simulink model "ES105A_StHlthSigNormn"  (R2013b)
settings: Solver=FixedStepDiscrete  SolverMode=SingleTasking  StartTime=0.0  StopTime=1  FixedStep=0.002  RelTol=1e-3
undefined symbols (not defined in the file): ARCHGLBPRM_FLOATZEROTHD_ULS_F32, CurrMeasCorrlnMaxErrCurr, CURRMOTSUMDIVBYZEROPROTNVAL_AMPR_F32, DIGTQDIVBYZEROPROTNVAL_HWNWTMTR_F32, DutyCycThermProtnDutyCycFildThd, EcuTMeasRngDiagcMax, EcuTMeasRngDiagcMin, EotLrngAuthyStrtLrn, FRICESTIMNDIVBYZEROPROTNVAL_HWNWTMTR_F32, HLTH0PERC_CNT_U08, HLTH100PERC_CNT_F32, HLTH100PERC_CNT_U08, HLTH50PERC_CNT_U08, HwTqCorrlnChATraSumSetFltThd, HwTqCorrlnChBTraSumSetFltThd, HWTQIDPTSIG_CNT_U08, MOTAG2MEAS_VALMAXERR_VOLTSQD_F32, MOTAG2MEAS_VALMINERR_VOLTSQD_F32, MOTAGCORRLN_MOTAGCORRLNERRTHD_MOTREVELEC_U0P16, MotDrvDiagcErrThd, MOTPOS2DIVBYZEROPROTNVAL2_VOLTSQD_F32, MOTPOS2DIVBYZEROPROTNVAL_VOLTSQD_F32, MOTPOSNERRDIVBYZEROPROTNVAL_MOTREV_U16, MOTPOSNERRZEROTHD_MOTREV_U0P16, NtcNr1, NtcSts1, PHAVLTGDIVBYZEROPROTNVAL_NANOSEC_F32, SigQlfr1, STHLTHSCAGFAC_CNT_F32, StHlthSigNormnAbsltMotPosDifStHlthDiagThd, StHlthSigNormnCurrMotSumStHlthDiagThd, StHlthSigNormnDigTqStHlthDiagThd, StHlthSigNormnDutyCycFltLimThd, StHlthSigNormnHiCtrlrT, StHlthSigNormnIdptSigStHlthSca, StHlthSigNormnLoCtrlrT, StHlthSigNormnMaxFricThd, StHlthSigNormnMinRackTrvlLim, StHlthSigNormnMotPosStHlthDiagThd, StHlthSigNormnMotVelCal, StHlthSigNormnPhaInfoStHlthDiagThd, StHlthSigNormnStHlthCorrlnErr, StHlthSigNormnStHlthCurrMotSum, StHlthSigNormnStHlthPhaInfo, StHlthSigNormnValMaxStHlthErr, StHlthSigNormnValMinStHlthErr, StHlthSigNormnWhlImbRejctnThd, SysGlbPrmMotPoleCnt, TSTHLTH0PERC_CNT_U08, u2, u3, u4, VLTGSTHLTH0PERC_CNT_U08
libraries: NxtrLim x39, simulink x33, NxtrAbslt x4
(part 1 of 10)
settings Model: Creator=PRAVEEND2  LastModifiedBy=DZ1YRM
settings SolverCC: AutoInsertRateTranBlk=on  InsertRTBMode=Always
settings DataIOCC: LimitDataPoints=off  SaveFormat=Structure  ReturnWorkspaceOutputs=on
settings OptimizationCC: BlockReduction=off  InlineParams=on  ZeroExternalMemoryAtStartup=off  ZeroInternalMemoryAtStartup=off  OptimizeModelRefInitCode=on  LifeSpan=1
settings DebuggingCC: SignalInfNanChecking=error  SignalRangeChecking=warning  UnderspecifiedInitializationDetection=Simplified  SolverPrmCheckMsg=error  InheritedTsInSrcMsg=error  DiscreteInheritContinuousMsg=error  SingleTaskRateTransMsg=error  TasksWithSamePriorityMsg=error  SigSpecEnsureSampleTimeMsg=error  CheckMatrixSingularityMsg=error  ParameterUnderflowMsg=error  ParameterPrecisionLossMsg=error  ParameterTunabilityLossMsg=error  FixptConstUnderflowMsg=warning  FixptConstOverflowMsg=warning  VectorMatrixConversionMsg=error  SignalLabelMismatchMsg=error  UnconnectedInputMsg=error  UnconnectedOutputMsg=error  UnconnectedLineMsg=error  SFcnCompatibilityMsg=error  UniqueDataStoreMsg=warning  BusObjectLabelMismatch=error  RootOutportRequireBusObject=error  AssertControl=DisableAll  ModelReferenceIOMsg=error  ModelReferenceVersionMismatchMessage=warning  ModelReferenceIOMismatchMessage=error  ModelReferenceCSMismatchMessage=warning  ModelReferenceDataLoggingMessage=error  StateNameClashWarn=warning  StrictBusMsg=ErrorOnBusTreatedAsVector  NonBusSignalsTreatedAsBus=error  SFUnexpectedBacktrackingDiag=error  SFInvalidInputDataAccessInChartInitDiag=error  SFNoUnconditionalDefaultTransitionDiag=error  SFTransitionOutsideNaturalParentDiag=error  SFUnconditionalTransitionShadowingDiag=error  SFUndirectedBroadcastEventsDiag=error
settings ModelReferenceCC: ModelReferenceNumInstancesAllowed=Single
settings RTWCC: SystemTargetFile=autosar.tlc  GenCodeOnly=on  TemplateMakefile=ert_default_tmf  Description=AUTOSAR  GenerateReport=on  ProcessScript=autosar_make_rtw_hook  LaunchReport=on
settings CodeAppCC: GenerateComments=off  IgnoreCustomStorageClasses=off  CustomSymbolStrType=$N$R$M  CustomSymbolStrBlkIO=$N$M  SimulinkBlockComments=off
settings STFCustomTargetCC: ParMdlRefBuildCompliant=on  CompOptLevelCompliant=on  IncludeMdlTerminateFcn=off  CombineOutputUpdateFcns=on  SuppressErrorStatus=on  ERTFirstTimeCompliant=on  ERTCustomFileBanners=on  SupportNonFinite=off  SupportComplex=off  SupportContinuousTime=off  SupportNonInlinedSFcns=off  MATLABClassNameForMDSCustomization=Simulink.SoftwareTarget.ERTCustomization  AutosarCompliant=on  GRTInterface=off  SystemTargetFile=autosar.tlc
settings ERTTargetCC: CodeReplacementLibrary=ANSI_C  ConcurrentExecutionCompliant=off  IncludeMdlTerminateFcn=off  SuppressErrorStatus=on  SupportNonFinite=off  SupportComplex=off  ModelStepFunctionPrototypeControlCompliant=off  CPPClassGenCompliant=off  AutosarCompliant=on  InlinedParameterPlacement=NonHierarchical  ERTCustomFileTemplate=example_file_process.tlc  EnableUserReplacementTypes=on

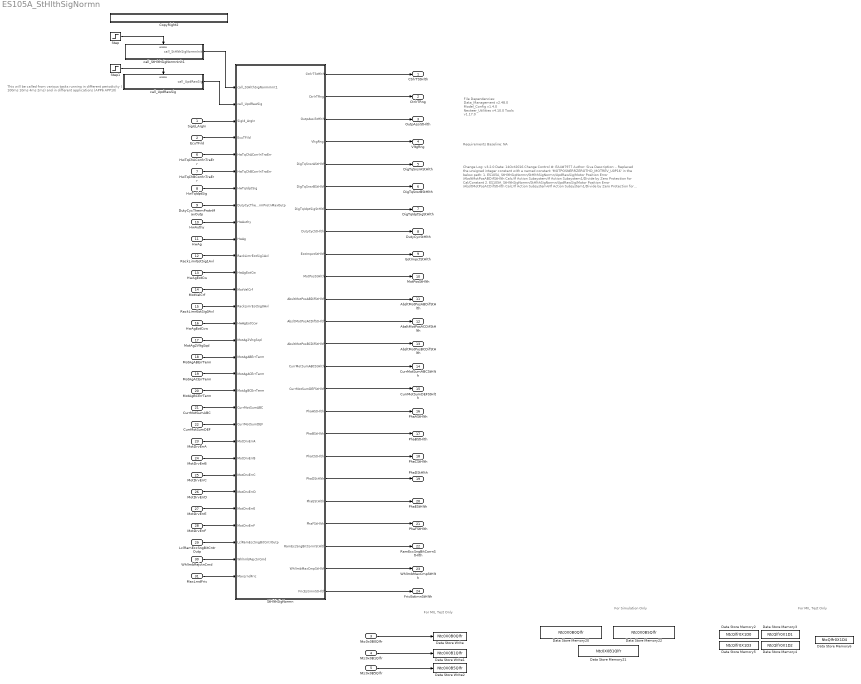
== system ES105A_StHlthSigNormn ==
  note: This will be called from various tasks running in different periodicity
      | ( 100ms 10ms 4ms 2ms) and in different applications (APP6 APP10)
  note: File Dependencies:
      |
      | Data_Management v2.48.0
      | Model_Config v1.4.0
      | Nexteer_Utilities v4.10.0
      | Tools v1.17.0
  note: Requirements Baseline: NA
  note: Change Log:
      |
      | v3.2.0
      | Date: 14Oct2016
      | Change Control #: EA4#7977
      | Author: Siva
      | Description:
      | - Replaced the unsigned integer constant with a named constant 'MOTPOSNERRZEROTHD_MOTREV_U0P16' in the below path:
      |         1. ES105A_StHlthSigNormn/StHlthSigNormn/UpdRawSig/Motor Position Error /AbsltMotPosABDifStHlth Calc/If Action
      |                Subsystem/If Action Subsystem1/Divide by Zero Protection for Cal/Constant
      |         2. ES105A_StHlthSigNormn/StHlthSigNormn/UpdRawSig/Motor Position Error /AbsltMotPosACDifStHlth Calc/If Action
      |                Subsystem4/If Action Subsystem1/Divide by Zero Protection for Cal/Constant1
      |         3. ES105A_StHlthSigNormn/StHlthSigNormn/UpdRawSig/Motor Position Error /AbsltMotPosBCDifStHlth Calc/If Action
      |                Subsystem8/If Action Subsystem1/Divide by Zero Protection for Cal/Constant1
      |
      | v3.1.0
      | Date: 28Sep2016
      | Change Control #: EA4#7764
      | Author: Siva
      | Description:
      | - Updated EOLFric (IRV signal) data dictionary information by swapping the ReadIn & WrittenIn attribute information.
      | - Updated Friction Estimation logic by performing all calculations in floating point mode and then converting it back to uint8 at the end.
      | - Removed extra saturation block present in the path(ES105A_StHlthSigNormn/StHlthSigNormn/UpdRawSig/Friction Estimation/LimStat_u2)
      |   as we have another saturation in the upstream logic.
      | - Replaced  'HLTH100PERC_CNT_U08' with a 'HLTH100PERC_CNT_F32' in both model & code.
      | - Replaced 'FRICESTSTHLTHLOLI_CNT_U08' & 'FRICESTSTHLTHHILI_CNT_U08' with 'FRICESTSTHLTHLOLI_CNT_F32' & 'FRICESTSTHLTHHILI_CNT_F32'
      |   in both model & code.
      | - Replaced numerical constant '1' of type 'uit8' with a 'float32' type.
      |
      | v3.0.0
      | Date: 23Sep2016
      | Change Control #: EA4#7256, EA4#7261, EA4#7303
      | Author: Siva
      | Description:
      | - Added Default labels to switch blocks in the below path:
      |        - ES105A_StHlthSigNormn/StHlthSigNormn/UpdRawSig/Switch Case1
      |        - ES105A_StHlthSigNormn/StHlthSigNormn/UpdRawSig/Digital Torque Sensor /Switch Case1
      |        - ES105A_StHlthSigNormn/StHlthSigNormn/UpdRawSig/Motor Position Error /Switch Case1
      |        - ES105A_StHlthSigNormn/StHlthSigNormn/UpdRawSig/Current Error/Switch Case1
      |        - ES105A_StHlthSigNormn/StHlthSigNormn/UpdRawSig/Phase Voltage Verification/Switch Case1
      | - Two New Outputs (WhlImbMaxCmpStHlth, FricEstimnStHlth) were added to model as well as DD.
      | - Two new Inputs (MaxLrndFric, WhlImbRejctnCmd) were added to to model and DD.
      |
      |
      |
      | v2.2.0
      | Date: 30Jun2016
      | Change Control #: EA4#5772, EA4#6242
      | Author: Siva, Mark Norman
      | Description:
      | - Added Saturation blocks to limit the Output value between [0 255] in all the below mentioned subsystems.
      |              -  Current Error
      |              -  Digital Torque Sensor
      |              -  Motor Position
      |              -  Motor Position Error
      |              -  Phase Voltage Verification
      | - Added Divide By Zero Protection blocks to limit the Output value between [0 255] in all the below mentioned subsystems.
      |              -  Motor Position
      | - Removed Default case from switch blocks in all the below mentioned subsystems.
      |              -  Current Error
      |              -  Digital Torque Sensor
      |              -  Motor Position Error
      |              -  Phase Voltage Verification
      |
      | Ver 2.1.0
      | DRW: Keyur G(KPIT)
      | Date:04-May-2016
      | CR- EA4#5550
      | -Default case added in switch cases to avoid simulation warnings
      | -Saturated input given to NTC status.
      | -Names of subsystems changed as per the requirement document.
      | -Name of signal 'VltgSqd' is changed to 'MotAg2VltgSqd' as it is an output from FDD ES241A. This change is done in model and .m file
      | - MotAgCorrlnErrThd and MOTAGCORRLN_MOTAGCORRLNERRTHD_MOTREVELEC_U0P16.LongName corrected
      | - Data type of Cal 'StHlthSigNormnStHlthCorrlnErr' is changed to u0p16 and 'StHlthSigNormnStHlthPhaInfo' is changed as float32
      | - Units of Cal StHlthSigNormnStHlthPhaInfo changed to 'NanoSec'
      | - Following constants have been added to replace magic numbers used for divide by zero protection logic
      | - DIGTQDIVBYZEROPROTNVAL_HWNWTMTR_F32, MOTPOSNERRDIVBYZEROPROTNVAL_MOTREV_U16, CURRMOTSUMDIVBYZEROPROTNVAL_AMPR_F32, PHAVLTGDIVBYZEROPROTNVAL_NANOSEC_F32
      | - Implementation added of PIM write and read for all NTC Sts calculations in Model and .m file.
      | - HUNDRED_CNT_U08 is changed to STHLTHSCAGFAC_CNT_F32.
      | - Removed Initialization of outputs from 'Init' function. Updated 'EngInit' and 'WrittenIn' field of all outputs with respective init value in Data Dict.
      | - Inside Digital Torque sensor Promotion of 1 is changed to Float32 in the below mentioned path:
      | 1).ES105A_StHlthSigNormn/StHlthSigNormn/UpdRawSig/Digital Torque Sensor /DigTqSnsrAStHlth Calc/If Action Subsystem1
      | 2) ES105A_StHlthSigNormn/StHlthSigNormn/UpdRawSig/Digital Torque Sensor /DigTqSnsrBStHlth Calc/If Action Subsystem3
      | - Inside EOT Impact Counter : HwAg comparion against zero is corrected to 'ARCHGLBPRM_FLOATZEROTHD_ULS_F32'
      | - Inside Motor Position Error in all cases: Divide-by-zero error protection logic Check against ARCHGLBPRM_FLOATZEROTHD_ULS_F32 is changed to zero.
      | - Initial output is kept hundred for all state health output port for all cases.
      | -Inside init subsystem, State Health PIM's are assigned with HLTH100PERC_CNT_U08 added
      |
      | Ver 2.0.0
      | DRW: Keyur G /Muragesh Asundi (KPIT)
      | Date:26-Apr-2016
      | CR- EA4#5550
      | -Design update as per new Requirements
      | -Constants for 0, 50,100 State of health is defined instead for having different constants for different State of health signals.
      | - Changes are marked with Red foreground color
      |
      | Ver 1.1.0
      | DRW:Praveen Devaraj(KPIT)
      | Date:11-Feb-2016
      | CR- EA4#3804
      | - Removed the PIM variable Intialization from Init function
      | -The Range limiter block placed outside the Init and server runnable is
      |   removed.Now it is placed inside the server runnable.
      | - In DD, EngValue are changed for EcuTMeasRngDiagcMax = 145,
      |   EcuTMeasRngDiagcMin = -45,StHlthSigNormnHiCtrlrT = 140
      |   StHlthSigNormnLoCtrlrT = -40.
      |
      | Ver: 1.0.0
      | DRW:Shradha Manusmare/Praveen Devaraj(KPIT)
      | Date:08-Feb-2016
      | CR- EA4#3077
      | - EA4 Initial Version
  note: For MIL Test Only
  note: For MIL Test Only
  note: For Simulation Only
  SigId_ArgIn : Inport
  EcuTFild : Inport  Port=2
  Ntc0x0B0Qlfr : Inport  Port=3
  Ntc0x0B1Qlfr : Inport  Port=4
  Ntc0x0B5Qlfr : Inport  Port=5
  HwTqChACorrlnTraErr : Inport  Port=6
  HwTqChBCorrlnTraErr : Inport  Port=7
  HwTqIdptSig : Inport  Port=8
  DutyCycThermProtnMaxOutp : Inport  Port=9
  HwAuthy : Inport  Port=10
  HwAg : Inport  Port=11
  RackLimrEotSig1Avl : Inport  Port=12
  HwAgEotCw : Inport  Port=13
  MotVelCrf : Inport  Port=14
  RackLimrEotSig0Avl : Inport  Port=15
  HwAgEotCcw : Inport  Port=16
  MotAg2VltgSqd : Inport  Port=17
  MotAgABErrTerm : Inport  Port=18
  MotAgACErrTerm : Inport  Port=19
  MotAgBCErrTerm : Inport  Port=20
  CurrMotSumABC : Inport  Port=21
  CurrMotSumDEF : Inport  Port=22
  MotDrvErrA : Inport  Port=23
  MotDrvErrB : Inport  Port=24
  MotDrvErrC : Inport  Port=25
  MotDrvErrD : Inport  Port=26
  MotDrvErrE : Inport  Port=27
  MotDrvErrF : Inport  Port=28
  LclRamEccSngBitCntrOutp : Inport  Port=29
  WhlImbRejctnCmd : Inport  Port=30
  MaxLrndFric : Inport  Port=31
  CopyRight2 : Subsystem  Description=|  mask(Copyright Information){none=on}
      | Copyright info block.                                               
      |                                                                     
      | Place copyright information at the top of every subsystem in design.
      mask prompts: none "No parameters"
      mask help: Place copyright information at the top of every subsystem in design.
      mask Display:
      | NxtrConf = 'Nexteer Confidential';
      | 
      | sys = bdroot; %handle for the current model ("system")
      | first = get_param(sys,'Created');
      | first = first(end-3:end);  %year is last four digits
      | 
      | last = get_param(sys,'LastModifiedDate');
      | if isempty(last)
      |     last = datestr(now,'yyyy');
      | else
      |     last = last(end-3:end);
      | end
      | 
      | if strcmp(first,last)
      |     fprintf('%s -- Copyright %s Nexteer',NxtrConf,first)
      | else
      |     fprintf('%s -- %s%s- %s Nexteer',NxtrConf,char(169),first,last)
      | end
  Data Store Memory2 : DataStoreMemory  DataStoreName=NtcQlfr0X1D0
  Data Store Memory20 : DataStoreMemory  DataStoreName=Ntc0X0B0Qlfr  InitialValue=SigQlfr1.SIGQLFR_NORES  OutDataTypeStr=Enum: SigQlfr1
      settings: LockScale=on
  Data Store Memory21 : DataStoreMemory  DataStoreName=Ntc0X0B1Qlfr  InitialValue=SigQlfr1.SIGQLFR_NORES  OutDataTypeStr=Enum: SigQlfr1
  Data Store Memory22 : DataStoreMemory  DataStoreName=Ntc0X0B5Qlfr  InitialValue=SigQlfr1.SIGQLFR_NORES  OutDataTypeStr=Enum: SigQlfr1
  Data Store Memory3 : DataStoreMemory  DataStoreName=NtcQlfr0X1D1
  Data Store Memory4 : DataStoreMemory  DataStoreName=NtcQlfr0X1D2
  Data Store Memory5 : DataStoreMemory  DataStoreName=NtcQlfr0X1D3
  Data Store Memory6 : DataStoreMemory  DataStoreName=NtcQlfr0X1D4
  Data Store Write : DataStoreWrite  DataStoreName=Ntc0X0B0Qlfr
  Data Store Write1 : DataStoreWrite  DataStoreName=Ntc0X0B1Qlfr
  Data Store Write2 : DataStoreWrite  DataStoreName=Ntc0X0B5Qlfr
  StHlthSigNormn : Subsystem  RequirementInfo={'linktype_rmi_doors' '0001022c (/ESG Group/FDD Module Requirements/EA4 Specific/ES105A_StHlthSigNormn)' '#ES105A_6' 'true' 'REQ: ES105A_6' '' ; 'linktype_rmi_doors' '0001022c (/ESG Group/FDD Module Requirements/EA4 Specific/ES105A_StHlthSigNormn)' '#ES105A_7' 'true' 'REQ: ES105A_7' '' } %GIDa_6ff4320a_4d8a_4175_a33b_02dee4a007dc
  Step : Step  Before=1  After=0  SampleTime=0.002
  Step1 : Step  SampleTime=0.002
  call_StHlthSigNormnInit1 : Subsystem  TreatAsAtomicUnit=on
  call_UpdRawSig : Subsystem  RequirementInfo={'linktype_rmi_doors' '0001022c (/ESG Group/FDD Module Requirements/EA4 Specific/ES105A_StHlthSigNormn)' '#ES105A_8' 'true' 'REQ: ES105A_8' '' } %GIDa_42dfbf7d_1872_4f82_ac73_93b666af75d7  TreatAsAtomicUnit=on
  CtrlrTStHlth : Outport
  CtrlrTRng : Outport  Port=2
  OutpAssiStHlth : Outport  Port=3
  VltgRng : Outport  Port=4
  DigTqSnsrAStHlth : Outport  Port=5
  DigTqSnsrBStHlth : Outport  Port=6
  DigTqIdptSigStHlth : Outport  Port=7
  DutyCycStHlth : Outport  Port=8
  EotImpctStHlth : Outport  Port=9
  MotPosStHlth : Outport  Port=10
  AbsltMotPosABDifStHlth : Outport  Port=11
  AbsltMotPosACDifStHlth : Outport  Port=12
  AbsltMotPosBCDifStHlth : Outport  Port=13
  CurrMotSumABCStHlth : Outport  Port=14
  CurrMotSumDEFStHlth : Outport  Port=15
  PhaAStHlth : Outport  Port=16
  PhaBStHlth : Outport  Port=17
  PhaCStHlth : Outport  Port=18
  PhaDStHlth : Outport  Port=19
  PhaEStHlth : Outport  Port=20
  PhaFStHlth : Outport  Port=21
  RamEccSngBitCorrnStHlth : Outport  Port=22
  WhlImbMaxCmpStHlth : Outport  Port=23
  FricEstimnStHlth : Outport  Port=24
  wires:
  Step/1 -> call_StHlthSigNormnInit1/Enable
  call_StHlthSigNormnInit1/1(call_StHlthSigNormnInit1) -> StHlthSigNormn/1(call_StHlthSigNormnInit1)
  call_UpdRawSig/1(call_UpdRawSig) -> StHlthSigNormn/2(call_UpdRawSig)
  Step1/1 -> call_UpdRawSig/Enable
  SigId_ArgIn/1 -> StHlthSigNormn/3(SigId_ArgIn)
  EcuTFild/1 -> StHlthSigNormn/4(EcuTFild)
  Ntc0x0B0Qlfr/1 -> Data Store Write/1
  Ntc0x0B1Qlfr/1 -> Data Store Write1/1
  Ntc0x0B5Qlfr/1 -> Data Store Write2/1
  DutyCycThermProtnMaxOutp/1 -> StHlthSigNormn/8(DutyCycThermProtnMaxOutp)
  HwTqChACorrlnTraErr/1 -> StHlthSigNormn/5(HwTqChACorrlnTraErr)
  HwTqIdptSig/1 -> StHlthSigNormn/7(HwTqIdptSig)
  HwTqChBCorrlnTraErr/1 -> StHlthSigNormn/6(HwTqChBCorrlnTraErr)
  HwAuthy/1 -> StHlthSigNormn/9(HwAuthy)
  HwAg/1 -> StHlthSigNormn/10(HwAg)
  RackLimrEotSig1Avl/1 -> StHlthSigNormn/11(RackLimrEotSig1Avl)
  HwAgEotCw/1 -> StHlthSigNormn/12(HwAgEotCw)
  MotVelCrf/1 -> StHlthSigNormn/13(MotVelCrf)
  RackLimrEotSig0Avl/1 -> StHlthSigNormn/14(RackLimrEotSig0Avl)
  HwAgEotCcw/1 -> StHlthSigNormn/15(HwAgEotCcw)
  MotAg2VltgSqd/1 -> StHlthSigNormn/16(MotAg2VltgSqd)
  MotAgABErrTerm/1 -> StHlthSigNormn/17(MotAgABErrTerm)
  MotAgACErrTerm/1 -> StHlthSigNormn/18(MotAgACErrTerm)
  MotAgBCErrTerm/1 -> StHlthSigNormn/19(MotAgBCErrTerm)
  CurrMotSumABC/1 -> StHlthSigNormn/20(CurrMotSumABC)
  LclRamEccSngBitCntrOutp/1 -> StHlthSigNormn/28(LclRamEccSngBitCntrOutp)
  MotDrvErrF/1 -> StHlthSigNormn/27(MotDrvErrF)
  MotDrvErrE/1 -> StHlthSigNormn/26(MotDrvErrE)
  MotDrvErrD/1 -> StHlthSigNormn/25(MotDrvErrD)
  MotDrvErrC/1 -> StHlthSigNormn/24(MotDrvErrC)
  MotDrvErrA/1 -> StHlthSigNormn/22(MotDrvErrA)
  CurrMotSumDEF/1 -> StHlthSigNormn/21(CurrMotSumDEF)
  MotDrvErrB/1 -> StHlthSigNormn/23(MotDrvErrB)
  MaxLrndFric/1 -> StHlthSigNormn/30(MaxLrndFric)
  WhlImbRejctnCmd/1 -> StHlthSigNormn/29(WhlImbRejctnCmd)
  StHlthSigNormn/22(RamEccSngBitCorrnStHlth) -> RamEccSngBitCorrnStHlth/1
  StHlthSigNormn/21(PhaFStHlth) -> PhaFStHlth/1
  StHlthSigNormn/20(PhaEStHlth) -> PhaEStHlth/1
  StHlthSigNormn/23(WhlImbMaxCmpStHlth) -> WhlImbMaxCmpStHlth/1
  StHlthSigNormn/24(FricEstimnStHlth) -> FricEstimnStHlth/1
  StHlthSigNormn/19(PhaDStHlth) -> PhaDStHlth/1
  StHlthSigNormn/18(PhaCStHlth) -> PhaCStHlth/1
  StHlthSigNormn/17(PhaBStHlth) -> PhaBStHlth/1
  StHlthSigNormn/16(PhaAStHlth) -> PhaAStHlth/1
  StHlthSigNormn/15(CurrMotSumDEFStHlth) -> CurrMotSumDEFStHlth/1
  StHlthSigNormn/14(CurrMotSumABCStHlth) -> CurrMotSumABCStHlth/1
  StHlthSigNormn/13(AbsltMotPosBCDifStHlth) -> AbsltMotPosBCDifStHlth/1
  StHlthSigNormn/12(AbsltMotPosACDifStHlth) -> AbsltMotPosACDifStHlth/1
  StHlthSigNormn/11(AbsltMotPosABDifStHlth) -> AbsltMotPosABDifStHlth/1
  StHlthSigNormn/10(MotPosStHlth) -> MotPosStHlth/1
  StHlthSigNormn/9(EotImpctStHlth) -> EotImpctStHlth/1
  StHlthSigNormn/8(DutyCycStHlth) -> DutyCycStHlth/1
  StHlthSigNormn/7(DigTqIdptSigStHlth) -> DigTqIdptSigStHlth/1
  StHlthSigNormn/6(DigTqSnsrBStHlth) -> DigTqSnsrBStHlth/1
  StHlthSigNormn/5(DigTqSnsrAStHlth) -> DigTqSnsrAStHlth/1
  StHlthSigNormn/4(VltgRng) -> VltgRng/1
  StHlthSigNormn/3(OutpAssiStHlth) -> OutpAssiStHlth/1
  StHlthSigNormn/2(CtrlrTRng) -> CtrlrTRng/1
  StHlthSigNormn/1(CtrlrTStHlth) -> CtrlrTStHlth/1

== system ES105A_StHlthSigNormn/CopyRight2 ==

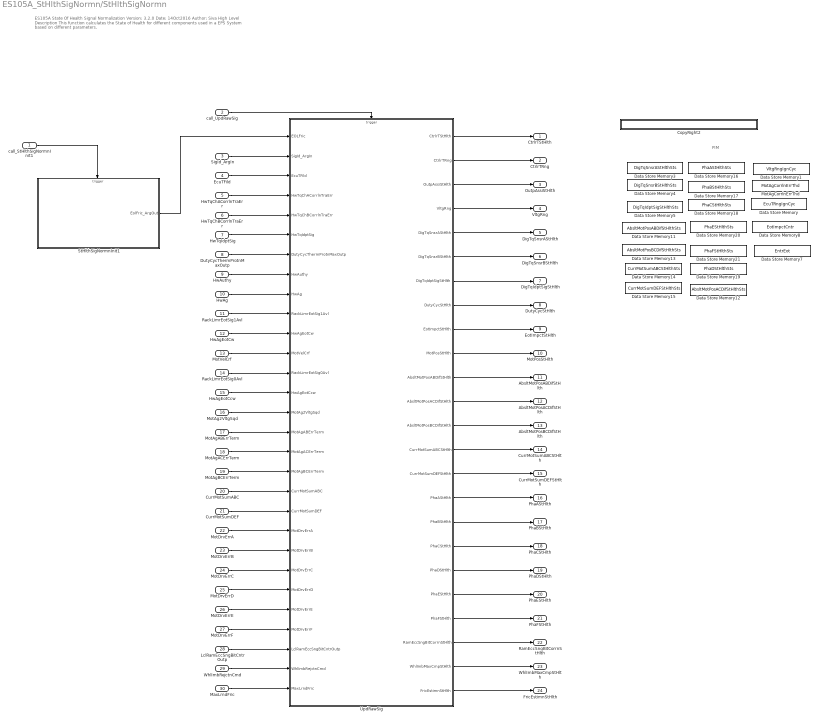
== system ES105A_StHlthSigNormn/StHlthSigNormn ==
  note: ES105A  State Of Health Signal Normalization
      |
      | Version: 3.2.0
      | Date: 14Oct2016
      |
      | Author: Siva
      |
      |
      | High Level Description
      |      This function calculates the State of Health for different components used in a EPS System based on different parameters.
  note: PIM
  call_StHlthSigNormnInit1 : Inport
  call_UpdRawSig : Inport  Port=2
  SigId_ArgIn : Inport  Port=3
  EcuTFild : Inport  RequirementInfo={'linktype_rmi_doors' '0001022c (/ESG Group/FDD Module Requirements/EA4 Specific/ES105A_StHlthSigNormn)' '#ES105A_14' 'true' 'REQ: ES105A_14' '' } %GIDa_49447a9e_c422_403c_bc64_e6d6f4ec146f  Port=4
  HwTqChACorrlnTraErr : Inport  Port=5
  HwTqChBCorrlnTraErr : Inport  Port=6
  HwTqIdptSig : Inport  Port=7
  DutyCycThermProtnMaxOutp : Inport  Port=8
  HwAuthy : Inport  Port=9
  HwAg : Inport  Port=10
  RackLimrEotSig1Avl : Inport  Port=11
  HwAgEotCw : Inport  Port=12
  MotVelCrf : Inport  Port=13
  RackLimrEotSig0Avl : Inport  Port=14
  HwAgEotCcw : Inport  Port=15
  MotAg2VltgSqd : Inport  Port=16
  MotAgABErrTerm : Inport  Port=17
  MotAgACErrTerm : Inport  Port=18
  MotAgBCErrTerm : Inport  Port=19
  CurrMotSumABC : Inport  Port=20
  CurrMotSumDEF : Inport  Port=21
  MotDrvErrA : Inport  Port=22
  MotDrvErrB : Inport  Port=23
  MotDrvErrC : Inport  Port=24
  MotDrvErrD : Inport  Port=25
  MotDrvErrE : Inport  Port=26
  MotDrvErrF : Inport  Port=27
  LclRamEccSngBitCntrOutp : Inport  Port=28
  WhlImbRejctnCmd : Inport  Port=29
  MaxLrndFric : Inport  Port=30
  CopyRight2 : Subsystem  Description=|  mask(Copyright Information){none=on}
      | Copyright info block.                                               
      |                                                                     
      | Place copyright information at the top of every subsystem in design.
      mask prompts: none "No parameters"
      mask help: Place copyright information at the top of every subsystem in design.
      mask Display:
      | NxtrConf = 'Nexteer Confidential';
      | 
      | sys = bdroot; %handle for the current model ("system")
      | first = get_param(sys,'Created');
      | first = first(end-3:end);  %year is last four digits
      | 
      | last = get_param(sys,'LastModifiedDate');
      | if isempty(last)
      |     last = datestr(now,'yyyy');
      | else
      |     last = last(end-3:end);
      | end
      | 
      | if strcmp(first,last)
      |     fprintf('%s -- Copyright %s Nexteer',NxtrConf,first)
      | else
      |     fprintf('%s -- %s%s- %s Nexteer',NxtrConf,char(169),first,last)
      | end
  Data Store Memory : DataStoreMemory  DataStoreName=EcuTRngIgnCyc  StateMustResolveToSignalObject=on
  Data Store Memory1 : DataStoreMemory  DataStoreName=VltgRngIgnCyc  StateMustResolveToSignalObject=on
  Data Store Memory11 : DataStoreMemory  DataStoreName=AbsltMotPosABDifStHlthSts  ReadBeforeWriteMsg=warning  WriteAfterWriteMsg=warning  WriteAfterReadMsg=warning  StateMustResolveToSignalObject=on
  Data Store Memory12 : DataStoreMemory  DataStoreName=AbsltMotPosACDifStHlthSts  ReadBeforeWriteMsg=warning  WriteAfterWriteMsg=warning  WriteAfterReadMsg=warning  StateMustResolveToSignalObject=on
  Data Store Memory13 : DataStoreMemory  DataStoreName=AbsltMotPosBCDifStHlthSts  ReadBeforeWriteMsg=warning  WriteAfterWriteMsg=warning  WriteAfterReadMsg=warning  StateMustResolveToSignalObject=on
  Data Store Memory14 : DataStoreMemory  DataStoreName=CurrMotSumABCStHlthSts  ReadBeforeWriteMsg=warning  WriteAfterWriteMsg=warning  WriteAfterReadMsg=warning  StateMustResolveToSignalObject=on
  Data Store Memory15 : DataStoreMemory  DataStoreName=CurrMotSumDEFStHlthSts  ReadBeforeWriteMsg=warning  WriteAfterWriteMsg=warning  WriteAfterReadMsg=warning  StateMustResolveToSignalObject=on
  Data Store Memory16 : DataStoreMemory  DataStoreName=PhaAStHlthSts  ReadBeforeWriteMsg=warning  WriteAfterWriteMsg=warning  WriteAfterReadMsg=warning  StateMustResolveToSignalObject=on
  Data Store Memory17 : DataStoreMemory  DataStoreName=PhaBStHlthSts  ReadBeforeWriteMsg=warning  WriteAfterWriteMsg=warning  WriteAfterReadMsg=warning  StateMustResolveToSignalObject=on
  Data Store Memory18 : DataStoreMemory  DataStoreName=PhaCStHlthSts  ReadBeforeWriteMsg=warning  WriteAfterWriteMsg=warning  WriteAfterReadMsg=warning  StateMustResolveToSignalObject=on
  Data Store Memory19 : DataStoreMemory  DataStoreName=PhaDStHlthSts  ReadBeforeWriteMsg=warning  WriteAfterWriteMsg=warning  WriteAfterReadMsg=warning  StateMustResolveToSignalObject=on
  Data Store Memory20 : DataStoreMemory  DataStoreName=PhaEStHlthSts  ReadBeforeWriteMsg=warning  WriteAfterWriteMsg=warning  WriteAfterReadMsg=warning  StateMustResolveToSignalObject=on
  Data Store Memory21 : DataStoreMemory  DataStoreName=PhaFStHlthSts  ReadBeforeWriteMsg=warning  WriteAfterWriteMsg=warning  WriteAfterReadMsg=warning  StateMustResolveToSignalObject=on
  Data Store Memory3 : DataStoreMemory  DataStoreName=DigTqSnsrAStHlthSts  ReadBeforeWriteMsg=warning  WriteAfterWriteMsg=warning  WriteAfterReadMsg=warning  StateMustResolveToSignalObject=on
  Data Store Memory4 : DataStoreMemory  DataStoreName=DigTqSnsrBStHlthSts  ReadBeforeWriteMsg=warning  WriteAfterWriteMsg=warning  WriteAfterReadMsg=warning  StateMustResolveToSignalObject=on
  Data Store Memory5 : DataStoreMemory  DataStoreName=DigTqIdptSigStHlthSts  ReadBeforeWriteMsg=warning  WriteAfterWriteMsg=warning  WriteAfterReadMsg=warning  StateMustResolveToSignalObject=on
  Data Store Memory7 : DataStoreMemory  DataStoreName=EntrEot  ReadBeforeWriteMsg=warning  WriteAfterWriteMsg=warning  WriteAfterReadMsg=warning  StateMustResolveToSignalObject=on
  Data Store Memory8 : DataStoreMemory  DataStoreName=EotImpctCntr  ReadBeforeWriteMsg=warning  WriteAfterWriteMsg=warning  WriteAfterReadMsg=warning  InitialValue=[]  StateMustResolveToSignalObject=on
  MotAgCorrlnErrThd : DataStoreMemory  Priority=0  DataStoreName=MotAgCorrlnErrThd  StateMustResolveToSignalObject=on
  StHlthSigNormnInit1 : Subsystem  RequirementInfo={'linktype_rmi_doors' '0001022c (/ESG Group/FDD Module Requirements/EA4 Specific/ES105A_StHlthSigNormn)' '#ES105A_9' 'true' 'REQ: ES105A_9' '' } %GIDa_bead402a_6bb2_4a86_9345_52509e5d4e33  TreatAsAtomicUnit=on
  UpdRawSig : Subsystem
  CtrlrTStHlth : Outport  RequirementInfo={'linktype_rmi_doors' '0001022c (/ESG Group/FDD Module Requirements/EA4 Specific/ES105A_StHlthSigNormn)' '#ES105A_26' 'true' 'REQ: ES105A_26' '' } %GIDa_65c3929a_51bb_49c3_afb4_64b9773c7714
  CtrlrTRng : Outport  RequirementInfo={'linktype_rmi_doors' '0001022c (/ESG Group/FDD Module Requirements/EA4 Specific/ES105A_StHlthSigNormn)' '#ES105A_26' 'true' 'REQ: ES105A_26' '' } %GIDa_a95003b5_b445_43be_bc6a_73ebe3208c85  Port=2
  OutpAssiStHlth : Outport  RequirementInfo={'linktype_rmi_doors' '0001022c (/ESG Group/FDD Module Requirements/EA4 Specific/ES105A_StHlthSigNormn)' '#ES105A_27' 'true' 'REQ: ES105A_27' '' } %GIDa_e353623f_856a_448e_be29_9e3993fbb0c1  Port=3
  VltgRng : Outport  RequirementInfo={'linktype_rmi_doors' '0001022c (/ESG Group/FDD Module Requirements/EA4 Specific/ES105A_StHlthSigNormn)' '#ES105A_27' 'true' 'REQ: ES105A_27' '' } %GIDa_05a6fd54_b3c2_4a26_803e_604d93a16994  Port=4
  DigTqSnsrAStHlth : Outport  Port=5
  DigTqSnsrBStHlth : Outport  Port=6
  DigTqIdptSigStHlth : Outport  Port=7
  DutyCycStHlth : Outport  Port=8
  EotImpctStHlth : Outport  Port=9
  MotPosStHlth : Outport  Port=10
  AbsltMotPosABDifStHlth : Outport  Port=11
  AbsltMotPosACDifStHlth : Outport  Port=12
  AbsltMotPosBCDifStHlth : Outport  Port=13
  CurrMotSumABCStHlth : Outport  Port=14
  CurrMotSumDEFStHlth : Outport  Port=15
  PhaAStHlth : Outport  Port=16
  PhaBStHlth : Outport  Port=17
  PhaCStHlth : Outport  Port=18
  PhaDStHlth : Outport  Port=19
  PhaEStHlth : Outport  Port=20
  PhaFStHlth : Outport  Port=21
  RamEccSngBitCorrnStHlth : Outport  Port=22
  WhlImbMaxCmpStHlth : Outport  Port=23
  FricEstimnStHlth : Outport  Port=24
  wires:
  call_StHlthSigNormnInit1/1 -> StHlthSigNormnInit1/Trigger
  UpdRawSig/21(PhaFStHlth) -> PhaFStHlth/1
  UpdRawSig/20(PhaEStHlth) -> PhaEStHlth/1
  UpdRawSig/22(RamEccSngBitCorrnStHlth) -> RamEccSngBitCorrnStHlth/1
  UpdRawSig/24(FricEstimnStHlth) -> FricEstimnStHlth/1
  UpdRawSig/23(WhlImbMaxCmpStHlth) -> WhlImbMaxCmpStHlth/1
  UpdRawSig/19(PhaDStHlth) -> PhaDStHlth/1
  UpdRawSig/18(PhaCStHlth) -> PhaCStHlth/1
  UpdRawSig/17(PhaBStHlth) -> PhaBStHlth/1
  UpdRawSig/16(PhaAStHlth) -> PhaAStHlth/1
  UpdRawSig/15(CurrMotSumDEFStHlth) -> CurrMotSumDEFStHlth/1
  UpdRawSig/14(CurrMotSumABCStHlth) -> CurrMotSumABCStHlth/1
  UpdRawSig/13(AbsltMotPosBCDifStHlth) -> AbsltMotPosBCDifStHlth/1
  UpdRawSig/12(AbsltMotPosACDifStHlth) -> AbsltMotPosACDifStHlth/1
  UpdRawSig/11(AbsltMotPosABDifStHlth) -> AbsltMotPosABDifStHlth/1
  UpdRawSig/10(MotPosStHlth) -> MotPosStHlth/1
  UpdRawSig/9(EotImpctStHlth) -> EotImpctStHlth/1
  UpdRawSig/8(DutyCycStHlth) -> DutyCycStHlth/1
  UpdRawSig/7(DigTqIdptSigStHlth) -> DigTqIdptSigStHlth/1
  UpdRawSig/6(DigTqSnsrBStHlth) -> DigTqSnsrBStHlth/1
  UpdRawSig/5(DigTqSnsrAStHlth) -> DigTqSnsrAStHlth/1
  UpdRawSig/4(VltgRng) -> VltgRng/1
  UpdRawSig/3(OutpAssiStHlth) -> OutpAssiStHlth/1
  UpdRawSig/2(CtrlrTRng) -> CtrlrTRng/1
  UpdRawSig/1(CtrlrTStHlth) -> CtrlrTStHlth/1
  call_UpdRawSig/1 -> UpdRawSig/Trigger
  MotDrvErrC/1 -> UpdRawSig/23(MotDrvErrC)
  MotDrvErrB/1 -> UpdRawSig/22(MotDrvErrB)
  MotDrvErrD/1 -> UpdRawSig/24(MotDrvErrD)
  MotDrvErrA/1 -> UpdRawSig/21(MotDrvErrA)
  MotDrvErrE/1 -> UpdRawSig/25(MotDrvErrE)
  CurrMotSumDEF/1 -> UpdRawSig/20(CurrMotSumDEF)
  MotDrvErrF/1 -> UpdRawSig/26(MotDrvErrF)
  MaxLrndFric/1 -> UpdRawSig/29(MaxLrndFric)
  CurrMotSumABC/1 -> UpdRawSig/19(CurrMotSumABC)
  LclRamEccSngBitCntrOutp/1 -> UpdRawSig/27(LclRamEccSngBitCntrOutp)
  WhlImbRejctnCmd/1 -> UpdRawSig/28(WhlImbRejctnCmd)
  MotAgBCErrTerm/1 -> UpdRawSig/18(MotAgBCErrTerm)
  MotAgACErrTerm/1 -> UpdRawSig/17(MotAgACErrTerm)
  MotAgABErrTerm/1 -> UpdRawSig/16(MotAgABErrTerm)
  MotAg2VltgSqd/1 -> UpdRawSig/15(MotAg2VltgSqd)
  HwAgEotCcw/1 -> UpdRawSig/14(HwAgEotCcw)
  RackLimrEotSig0Avl/1 -> UpdRawSig/13(RackLimrEotSig0Avl)
  MotVelCrf/1 -> UpdRawSig/12(MotVelCrf)
  HwAgEotCw/1 -> UpdRawSig/11(HwAgEotCw)
  RackLimrEotSig1Avl/1 -> UpdRawSig/10(RackLimrEotSig1Avl)
  HwAg/1 -> UpdRawSig/9(HwAg)
  HwAuthy/1 -> UpdRawSig/8(HwAuthy)
  DutyCycThermProtnMaxOutp/1 -> UpdRawSig/7(DutyCycThermProtnMaxOutp)
  HwTqIdptSig/1 -> UpdRawSig/6(HwTqIdptSig)
  HwTqChBCorrlnTraErr/1 -> UpdRawSig/5(HwTqChBCorrlnTraErr)
  HwTqChACorrlnTraErr/1 -> UpdRawSig/4(HwTqChACorrlnTraErr)
  EcuTFild/1 -> UpdRawSig/3("EcuTFild ")
  SigId_ArgIn/1 -> UpdRawSig/2(SigId_ArgIn)
  StHlthSigNormnInit1/1(EolFric_ArgOut) -> UpdRawSig/1(EOLFric)

== system ES105A_StHlthSigNormn/call_StHlthSigNormnInit1 ==
  Enable : EnablePort
  CopyRight2 : Subsystem  Description=|  mask(Copyright Information){none=on}
      | Copyright info block.                                               
      |                                                                     
      | Place copyright information at the top of every subsystem in design.
      mask prompts: none "No parameters"
      mask help: Place copyright information at the top of every subsystem in design.
      mask Display:
      | NxtrConf = 'Nexteer Confidential';
      | 
      | sys = bdroot; %handle for the current model ("system")
      | first = get_param(sys,'Created');
      | first = first(end-3:end);  %year is last four digits
      | 
      | last = get_param(sys,'LastModifiedDate');
      | if isempty(last)
      |     last = datestr(now,'yyyy');
      | else
      |     last = last(end-3:end);
      | end
      | 
      | if strcmp(first,last)
      |     fprintf('%s -- Copyright %s Nexteer',NxtrConf,first)
      | else
      |     fprintf('%s -- %s%s- %s Nexteer',NxtrConf,char(169),first,last)
      | end
  "call_StHlthSigNormnInit " : simulink/Ports & Subsystems/Function-Call Generator  sample_time=0  numberOfIterations=1
  call_StHlthSigNormnInit1 : Outport
  wires:
  "call_StHlthSigNormnInit "/1 -> call_StHlthSigNormnInit1/1

== system ES105A_StHlthSigNormn/call_UpdRawSig ==
  Enable : EnablePort
  CopyRight2 : Subsystem  Description=|  mask(Copyright Information){none=on}
      | Copyright info block.                                               
      |                                                                     
      | Place copyright information at the top of every subsystem in design.
      mask prompts: none "No parameters"
      mask help: Place copyright information at the top of every subsystem in design.
      mask Display:
      | NxtrConf = 'Nexteer Confidential';
      | 
      | sys = bdroot; %handle for the current model ("system")
      | first = get_param(sys,'Created');
      | first = first(end-3:end);  %year is last four digits
      | 
      | last = get_param(sys,'LastModifiedDate');
      | if isempty(last)
      |     last = datestr(now,'yyyy');
      | else
      |     last = last(end-3:end);
      | end
      | 
      | if strcmp(first,last)
      |     fprintf('%s -- Copyright %s Nexteer',NxtrConf,first)
      | else
      |     fprintf('%s -- %s%s- %s Nexteer',NxtrConf,char(169),first,last)
      | end
  "call_UpdRawSig " : simulink/Ports & Subsystems/Function-Call Generator  sample_time=0  numberOfIterations=1
  call_UpdRawSig : Outport
  wires:
  "call_UpdRawSig "/1 -> call_UpdRawSig/1

== system ES105A_StHlthSigNormn/StHlthSigNormn/CopyRight2 ==

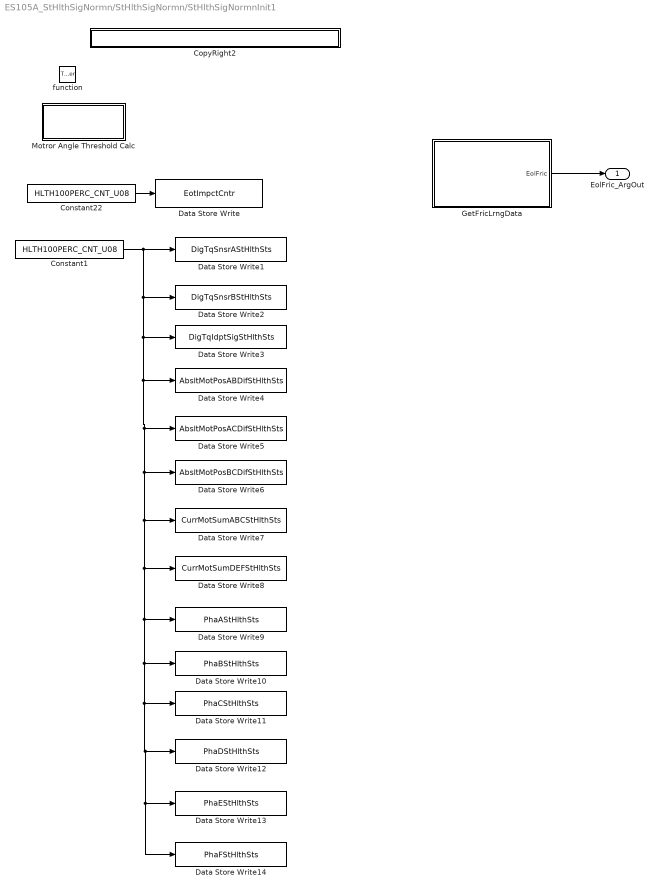
== system ES105A_StHlthSigNormn/StHlthSigNormn/StHlthSigNormnInit1 ==
  function : TriggerPort  TriggerType=function-call
  Constant1 : Constant  Value=HLTH100PERC_CNT_U08  OutDataTypeStr=uint8
  Constant22 : Constant  Value=HLTH100PERC_CNT_U08  OutDataTypeStr=uint8
  CopyRight2 : Subsystem  Description=|  mask(Copyright Information){none=on}
      | Copyright info block.                                               
      |                                                                     
      | Place copyright information at the top of every subsystem in design.
      mask prompts: none "No parameters"
      mask help: Place copyright information at the top of every subsystem in design.
      mask Display:
      | NxtrConf = 'Nexteer Confidential';
      | 
      | sys = bdroot; %handle for the current model ("system")
      | first = get_param(sys,'Created');
      | first = first(end-3:end);  %year is last four digits
      | 
      | last = get_param(sys,'LastModifiedDate');
      | if isempty(last)
      |     last = datestr(now,'yyyy');
      | else
      |     last = last(end-3:end);
      | end
      | 
      | if strcmp(first,last)
      |     fprintf('%s -- Copyright %s Nexteer',NxtrConf,first)
      | else
      |     fprintf('%s -- %s%s- %s Nexteer',NxtrConf,char(169),first,last)
      | end
  Data Store Write : DataStoreWrite  DataStoreName=EotImpctCntr
  Data Store Write1 : DataStoreWrite  DataStoreName=DigTqSnsrAStHlthSts
  Data Store Write10 : DataStoreWrite  DataStoreName=PhaBStHlthSts
  Data Store Write11 : DataStoreWrite  DataStoreName=PhaCStHlthSts
  Data Store Write12 : DataStoreWrite  DataStoreName=PhaDStHlthSts
  Data Store Write13 : DataStoreWrite  DataStoreName=PhaEStHlthSts
  Data Store Write14 : DataStoreWrite  DataStoreName=PhaFStHlthSts
  Data Store Write2 : DataStoreWrite  DataStoreName=DigTqSnsrBStHlthSts
  Data Store Write3 : DataStoreWrite  DataStoreName=DigTqIdptSigStHlthSts
  Data Store Write4 : DataStoreWrite  DataStoreName=AbsltMotPosABDifStHlthSts
  Data Store Write5 : DataStoreWrite  DataStoreName=AbsltMotPosACDifStHlthSts
  Data Store Write6 : DataStoreWrite  DataStoreName=AbsltMotPosBCDifStHlthSts
  Data Store Write7 : DataStoreWrite  DataStoreName=CurrMotSumABCStHlthSts
  Data Store Write8 : DataStoreWrite  DataStoreName=CurrMotSumDEFStHlthSts
  Data Store Write9 : DataStoreWrite  DataStoreName=PhaAStHlthSts
  GetFricLrngData : Subsystem
  Motror Angle Threshold Calc : Subsystem
  EolFric_ArgOut : Outport
  wires:
  Constant22/1 -> Data Store Write/1
  Constant1/1 -> Data Store Write9/1, Data Store Write10/1, Data Store Write11/1, Data Store Write12/1, Data Store Write13/1, Data Store Write14/1, Data Store Write8/1, Data Store Write7/1, Data Store Write6/1, Data Store Write5/1, Data Store Write4/1, Data Store Write3/1, Data Store Write2/1, Data Store Write1/1
  GetFricLrngData/1(EolFric) -> EolFric_ArgOut/1

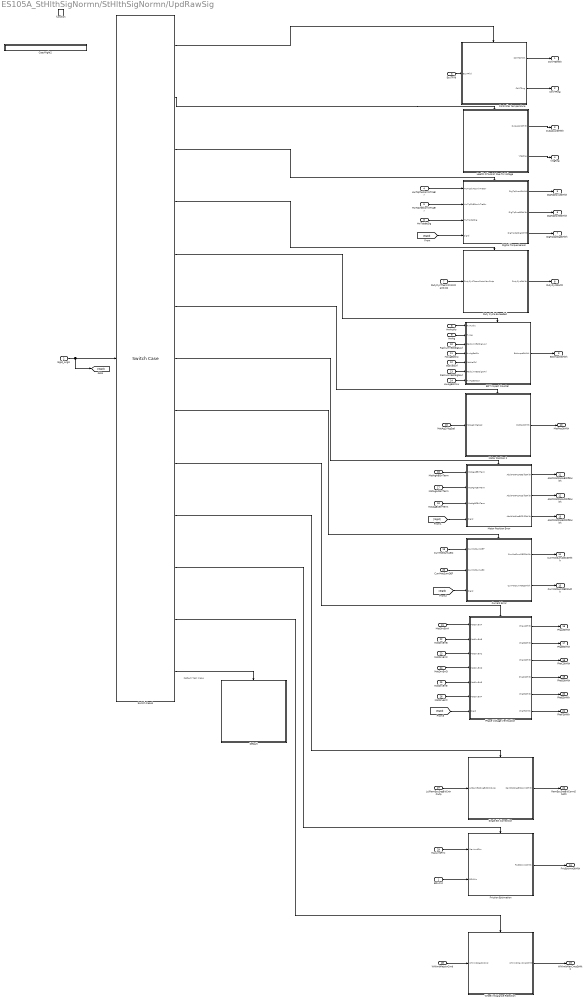
== system ES105A_StHlthSigNormn/StHlthSigNormn/UpdRawSig ==
  note: Default Test Case
  EOLFric : Inport
  SigId_ArgIn : Inport  Port=2
  "EcuTFild " : Inport  Port=3
  HwTqChACorrlnTraErr : Inport  Port=4
  HwTqChBCorrlnTraErr : Inport  Port=5
  HwTqIdptSig : Inport  Port=6
  DutyCycThermProtnMaxOutp : Inport  Port=7
  HwAuthy : Inport  Port=8
  HwAg : Inport  Port=9
  RackLimrEotSig1Avl : Inport  Port=10
  HwAgEotCw : Inport  Port=11
  MotVelCrf : Inport  Port=12
  RackLimrEotSig0Avl : Inport  Port=13
  HwAgEotCcw : Inport  Port=14
  MotAg2VltgSqd : Inport  Port=15
  MotAgABErrTerm : Inport  Port=16
  MotAgACErrTerm : Inport  Port=17
  MotAgBCErrTerm : Inport  Port=18
  CurrMotSumABC : Inport  Port=19
  CurrMotSumDEF : Inport  Port=20
  MotDrvErrA : Inport  Port=21
  MotDrvErrB : Inport  Port=22
  MotDrvErrC : Inport  Port=23
  MotDrvErrD : Inport  Port=24
  MotDrvErrE : Inport  Port=25
  MotDrvErrF : Inport  Port=26
  LclRamEccSngBitCntrOutp : Inport  Port=27
  WhlImbRejctnCmd : Inport  Port=28
  MaxLrndFric : Inport  Port=29
  function : TriggerPort  TriggerType=function-call
  " EOT Impact Counter" : Subsystem  RequirementInfo={'linktype_rmi_doors' '0001022c (/ESG Group/FDD Module Requirements/EA4 Specific/ES105A_StHlthSigNormn)' '#ES105A_48' 'true' 'REQ: ES105A_48' '' ; 'linktype_rmi_doors' '0001022c (/ESG Group/FDD Module Requirements/EA4 Specific/ES105A_StHlthSigNormn)' '#ES105A_49' 'true' 'REQ: ES105A_49' '' } %GIDa_91bcaadc_6e80_435e_b1cb_1267a6017c86
  " Health Of Assist Due To Voltage" : Subsystem  RequirementInfo={'linktype_rmi_doors' '0001022c (/ESG Group/FDD Module Requirements/EA4 Specific/ES105A_StHlthSigNormn)' '#ES105A_48' 'true' 'REQ: ES105A_48' '' ; 'linktype_rmi_doors' '0001022c (/ESG Group/FDD Module Requirements/EA4 Specific/ES105A_StHlthSigNormn)' '#ES105A_49' 'true' 'REQ: ES105A_49' '' } %GIDa_be3b1dd5_5c29_4513_8011_7bf0c154f42d
  Controller temperature : Subsystem  RequirementInfo={'linktype_rmi_doors' '0001022c (/ESG Group/FDD Module Requirements/EA4 Specific/ES105A_StHlthSigNormn)' '#ES105A_39' 'true' 'REQ: ES105A_39' '' ; 'linktype_rmi_doors' '0001022c (/ESG Group/FDD Module Requirements/EA4 Specific/ES105A_StHlthSigNormn)' '#ES105A_40' 'true' 'REQ: ES105A_40' '' } %GIDa_52b4cf45_595e_408d_a772_5a460695706a
  CopyRight2 : Subsystem  Description=|  mask(Copyright Information){none=on}
      | Copyright info block.                                               
      |                                                                     
      | Place copyright information at the top of every subsystem in design.
      mask prompts: none "No parameters"
      mask help: Place copyright information at the top of every subsystem in design.
      mask Display:
      | NxtrConf = 'Nexteer Confidential';
      | 
      | sys = bdroot; %handle for the current model ("system")
      | first = get_param(sys,'Created');
      | first = first(end-3:end);  %year is last four digits
      | 
      | last = get_param(sys,'LastModifiedDate');
      | if isempty(last)
      |     last = datestr(now,'yyyy');
      | else
      |     last = last(end-3:end);
      | end
      | 
      | if strcmp(first,last)
      |     fprintf('%s -- Copyright %s Nexteer',NxtrConf,first)
      | else
      |     fprintf('%s -- %s%s- %s Nexteer',NxtrConf,char(169),first,last)
      | end
  Current Error : Subsystem
  Default : Subsystem
  "Digital Torque Sensor " : Subsystem  RequirementInfo={'linktype_rmi_doors' '0001022c (/ESG Group/FDD Module Requirements/EA4 Specific/ES105A_StHlthSigNormn)' '#ES105A_48' 'true' 'REQ: ES105A_48' '' ; 'linktype_rmi_doors' '0001022c (/ESG Group/FDD Module Requirements/EA4 Specific/ES105A_StHlthSigNormn)' '#ES105A_49' 'true' 'REQ: ES105A_49' '' } %GIDa_59243a04_9943_4c27_90dd_fcb3f2a7a07f
  Duty Cycle Exceeded : Subsystem  RequirementInfo={'linktype_rmi_doors' '0001022c (/ESG Group/FDD Module Requirements/EA4 Specific/ES105A_StHlthSigNormn)' '#ES105A_48' 'true' 'REQ: ES105A_48' '' ; 'linktype_rmi_doors' '0001022c (/ESG Group/FDD Module Requirements/EA4 Specific/ES105A_StHlthSigNormn)' '#ES105A_49' 'true' 'REQ: ES105A_49' '' } %GIDa_942d087d_dfe4_428e_81ec_65c85e7dcb84
  Friction Estimation : Subsystem  RequirementInfo={'linktype_rmi_doors' '0001022c (/ESG Group/FDD Module Requirements/EA4 Specific/ES105A_StHlthSigNormn)' '#ES105A_48' 'true' 'REQ: ES105A_48' '' ; 'linktype_rmi_doors' '0001022c (/ESG Group/FDD Module Requirements/EA4 Specific/ES105A_StHlthSigNormn)' '#ES105A_49' 'true' 'REQ: ES105A_49' '' } %GIDa_0a357e03_a7d0_4d22_b80f_6f969b2d9eb5
  "Motor Position 2 " : Subsystem
  "Motor Position Error " : Subsystem
  Phase Voltage Verification : Subsystem
  "Single Bit Correction " : Subsystem
  Switch Case1 : SwitchCase  CaseConditions={StHlthMonSig3.STHLTHMONSIG_ECUTFILTD,StHlthMonSig3.STHLTHMONSIG_ASSIDUETOVLTG,[StHlthMonSig3.STHLTHMONSIG_DIGTQSNSRA,StHlthMonSig3.STHLTHMONSIG_DIGTQSNSRB,StHlthMonSig3.STHLTHMONSIG_DIGTQIDPTSIG],StHlthMonSig3.STHLTHMONSIG_DUTYCYC,StHlthMonSig3.STHLTHMONSIG_EOTIMPCT,StHlthMonSig3.STHLTHMONSIG_MOTPOS,[StHlthMonSig3.STHLTHMONSIG_MOTPOSABDIFF, StHlthMonSig3.STHLTHMONSIG_MOTPOSACDIFF,StHlthMonSig3.STHLTHMONSIG_MOTPOSBCDIFF],[StHlthMonSig3.STHLTHMONSIG_CURRMOTSUMABC,StHlthMonSig3.STHLTHMONSIG_CURRMOTSUMDEF],[StHlthMonSig3.STHLTHMONSIG_MOTPOSPHASEA,StHlthMonSig3.STHLTHMONSIG_MOTPOSPHASEB,StHlthMonSig3.STHLTHMONSIG_MOTPOSPHASEC,StHlthMonSig3.STHLTHMONSIG_MOTPOSPHASED,StHlthMonSig3.STHLTHMONSIG_MOTPOSPHASEE,StHlthMonSig3.STHLTHMONSIG_MOTPOSPHASEF],StHlthMonSig3.STHLTHMONSIG_BITCORRN,StHlthMonSig3.STHLTHMONSIG_FRICESTIMN,StHlthMonSig3.STHLTHMONSIG_WHLIMBREJCTN}
  Wheel Imbalance Rejection : Subsystem  RequirementInfo={'linktype_rmi_doors' '0001022c (/ESG Group/FDD Module Requirements/EA4 Specific/ES105A_StHlthSigNormn)' '#ES105A_48' 'true' 'REQ: ES105A_48' '' ; 'linktype_rmi_doors' '0001022c (/ESG Group/FDD Module Requirements/EA4 Specific/ES105A_StHlthSigNormn)' '#ES105A_49' 'true' 'REQ: ES105A_49' '' } %GIDa_a511e5d5_b560_4ef5_a57b_5839357b50d2
  CtrlrTStHlth : Outport  InitialOutput=HLTH100PERC_CNT_U08
      settings: AttributesFormatString=Initial Output: %<InitialOutput>
  CtrlrTRng : Outport  Port=2  InitialOutput=0
      settings: AttributesFormatString=Initial Output: %<InitialOutput>
  OutpAssiStHlth : Outport  Port=3  InitialOutput=HLTH100PERC_CNT_U08
      settings: AttributesFormatString=Initial Output: %<InitialOutput>
  VltgRng : Outport  Port=4  InitialOutput=0
      settings: AttributesFormatString=Initial Output: %<InitialOutput>
  DigTqSnsrAStHlth : Outport  Port=5  InitialOutput=HLTH100PERC_CNT_U08
      settings: AttributesFormatString=Initial Output: %<InitialOutput>
  DigTqSnsrBStHlth : Outport  Port=6  InitialOutput=HLTH100PERC_CNT_U08
      settings: AttributesFormatString=Initial Output: %<InitialOutput>
  DigTqIdptSigStHlth : Outport  Port=7  InitialOutput=HLTH100PERC_CNT_U08
      settings: AttributesFormatString=Initial Output: %<InitialOutput>
  DutyCycStHlth : Outport  Port=8  InitialOutput=HLTH100PERC_CNT_U08
      settings: AttributesFormatString=Initial Output: %<InitialOutput>
  EotImpctStHlth : Outport  Port=9  InitialOutput=HLTH100PERC_CNT_U08
      settings: AttributesFormatString=Initial Output: %<InitialOutput>
  MotPosStHlth : Outport  Port=10  InitialOutput=HLTH100PERC_CNT_U08
      settings: AttributesFormatString=Initial Output: %<InitialOutput>
  AbsltMotPosABDifStHlth : Outport  Port=11  InitialOutput=HLTH100PERC_CNT_U08
      settings: AttributesFormatString=Initial Output: %<InitialOutput>
  AbsltMotPosACDifStHlth : Outport  Port=12  InitialOutput=HLTH100PERC_CNT_U08
      settings: AttributesFormatString=Initial Output: %<InitialOutput>
  AbsltMotPosBCDifStHlth : Outport  Port=13  InitialOutput=HLTH100PERC_CNT_U08
      settings: AttributesFormatString=Initial Output: %<InitialOutput>
  CurrMotSumABCStHlth : Outport  Port=14  InitialOutput=HLTH100PERC_CNT_U08
      settings: AttributesFormatString=Initial Output: %<InitialOutput>
  CurrMotSumDEFStHlth : Outport  Port=15  InitialOutput=HLTH100PERC_CNT_U08
      settings: AttributesFormatString=Initial Output: %<InitialOutput>
  PhaAStHlth : Outport  Port=16  InitialOutput=HLTH100PERC_CNT_U08
      settings: AttributesFormatString=Initial Output: %<InitialOutput>
  PhaBStHlth : Outport  Port=17  InitialOutput=HLTH100PERC_CNT_U08
      settings: AttributesFormatString=Initial Output: %<InitialOutput>
  PhaCStHlth : Outport  Port=18  InitialOutput=HLTH100PERC_CNT_U08
      settings: AttributesFormatString=Initial Output: %<InitialOutput>
  PhaDStHlth : Outport  Port=19  InitialOutput=HLTH100PERC_CNT_U08
      settings: AttributesFormatString=Initial Output: %<InitialOutput>
  PhaEStHlth : Outport  Port=20  InitialOutput=HLTH100PERC_CNT_U08
      settings: AttributesFormatString=Initial Output: %<InitialOutput>
  PhaFStHlth : Outport  Port=21  InitialOutput=HLTH100PERC_CNT_U08
      settings: AttributesFormatString=Initial Output: %<InitialOutput>
  RamEccSngBitCorrnStHlth : Outport  Port=22  InitialOutput=HLTH100PERC_CNT_U08
      settings: AttributesFormatString=Initial Output: %<InitialOutput>
  WhlImbMaxCmpStHlth : Outport  Port=23
  FricEstimnStHlth : Outport  Port=24
  wires:
  Controller temperature/1(CtrlrTStHlth) -> CtrlrTStHlth/1
  " Health Of Assist Due To Voltage"/1(OutpAssiStHlth) -> OutpAssiStHlth/1
  SigId_ArgIn/1 -> [SigId], Switch Case1/1
  "EcuTFild "/1 -> Controller temperature/1(EcuTFild)
  Switch Case1/1 -> Controller temperature/Action
  Switch Case1/2 -> " Health Of Assist Due To Voltage"/Action
  Controller temperature/2(CtrlrTRng) -> CtrlrTRng/1
  " Health Of Assist Due To Voltage"/2(" VltgRng") -> VltgRng/1
  DutyCycThermProtnMaxOutp/1 -> Duty Cycle Exceeded/1(DutyCycThermProtnMaxOutp)
  Duty Cycle Exceeded/1(DutyCycStHlth) -> DutyCycStHlth/1
  HwAuthy/1 -> " EOT Impact Counter"/1("HwAuthy ")
  HwAg/1 -> " EOT Impact Counter"/2(HwAg)
  RackLimrEotSig0Avl/1 -> " EOT Impact Counter"/6(RackLimrEotSig0Avl)
  HwAgEotCw/1 -> " EOT Impact Counter"/4(HwAgEotCw)
  RackLimrEotSig1Avl/1 -> " EOT Impact Counter"/3(RackLimrEotSig1Avl)
  HwAgEotCcw/1 -> " EOT Impact Counter"/7(HwAgEotCcw)
  MotVelCrf/1 -> " EOT Impact Counter"/5(MotVelCrf)
  " EOT Impact Counter"/1(EotImpctStHlth) -> EotImpctStHlth/1
  MotAg2VltgSqd/1 -> "Motor Position 2 "/1(MotAg2VltgSqd)
  "Motor Position 2 "/1(MotPosStHlth) -> MotPosStHlth/1
  Current Error/1(CurrMotSumDEFStHlth) -> CurrMotSumABCStHlth/1
  LclRamEccSngBitCntrOutp/1 -> "Single Bit Correction "/1(LclRamEccSngBitCntrOutp)
  "Single Bit Correction "/1(RamEccSngBitCorrnStHlth) -> RamEccSngBitCorrnStHlth/1
  Switch Case1/3 -> "Digital Torque Sensor "/Action
  Switch Case1/4 -> Duty Cycle Exceeded/Action
  Switch Case1/5 -> " EOT Impact Counter"/Action
  Switch Case1/6 -> "Motor Position 2 "/Action
  Switch Case1/7 -> "Motor Position Error "/Action
  Switch Case1/8 -> Current Error/Action
  Switch Case1/9 -> Phase Voltage Verification/Action
  Switch Case1/10 -> "Single Bit Correction "/Action
  HwTqChACorrlnTraErr/1 -> "Digital Torque Sensor "/1(HwTqChACorrlnTraErr)
  HwTqChBCorrlnTraErr/1 -> "Digital Torque Sensor "/2(HwTqChBCorrlnTraErr)
  HwTqIdptSig/1 -> "Digital Torque Sensor "/3(HwTqIdptSig)
  [SigId] -> "Digital Torque Sensor "/4(SigId)
  "Digital Torque Sensor "/1(DigTqSnsrAStHlth) -> DigTqSnsrAStHlth/1
  "Digital Torque Sensor "/2(DigTqSnsrBStHlth) -> DigTqSnsrBStHlth/1
  "Digital Torque Sensor "/3(" DigTqIdptSigStHlth") -> DigTqIdptSigStHlth/1
  MotAgABErrTerm/1 -> "Motor Position Error "/1(MotAgABErrTerm)
  MotAgACErrTerm/1 -> "Motor Position Error "/2(MotAgACErrTerm)
  MotAgBCErrTerm/1 -> "Motor Position Error "/3(MotAgBCErrTerm)
  [SigId] -> "Motor Position Error "/4(SigId)
  "Motor Position Error "/1(AbsltMotPosABDifStHlth) -> AbsltMotPosABDifStHlth/1
  "Motor Position Error "/2(AbsltMotPosACDifStHlth) -> AbsltMotPosACDifStHlth/1
  "Motor Position Error "/3(AbsltMotPosBCDifStHlth) -> AbsltMotPosBCDifStHlth/1
  CurrMotSumABC/1 -> Current Error/1(CurrMotSumDEF)
  CurrMotSumDEF/1 -> Current Error/2(CurrMotSumABC)
  [SigId] -> Current Error/3(SigId)
  Current Error/2(CurrMotSumABCStHlth) -> CurrMotSumDEFStHlth/1
  Phase Voltage Verification/1(PhaAStHlth) -> PhaAStHlth/1
  Phase Voltage Verification/2(PhaBStHlth) -> PhaBStHlth/1
  Phase Voltage Verification/3(PhaCStHlth) -> PhaCStHlth/1
  Phase Voltage Verification/4(PhaDStHlth) -> PhaDStHlth/1
  Phase Voltage Verification/5(PhaEStHlth) -> PhaEStHlth/1
  Phase Voltage Verification/6(PhaFStHlth) -> PhaFStHlth/1
  MotDrvErrA/1 -> Phase Voltage Verification/1(MotDrvErrA)
  MotDrvErrB/1 -> Phase Voltage Verification/2(MotDrvErrB)
  MotDrvErrC/1 -> Phase Voltage Verification/3(MotDrvErrC)
  MotDrvErrD/1 -> Phase Voltage Verification/4(MotDrvErrD)
  MotDrvErrE/1 -> Phase Voltage Verification/5(MotDrvErrE)
  MotDrvErrF/1 -> Phase Voltage Verification/6(MotDrvErrF)
  [SigId] -> Phase Voltage Verification/7(SigId)
  Switch Case1/13 -> Default/Action
  WhlImbRejctnCmd/1 -> Wheel Imbalance Rejection/1(WhlImbRejctnCmd)
  Wheel Imbalance Rejection/1(WhlImbMaxCmpStHlth) -> WhlImbMaxCmpStHlth/1
  Switch Case1/11 -> Friction Estimation/Action
  Switch Case1/12 -> Wheel Imbalance Rejection/Action
  MaxLrndFric/1 -> Friction Estimation/1(MaxLrndFric)
  Friction Estimation/1(FricEstimnStHlth) -> FricEstimnStHlth/1
  EOLFric/1 -> Friction Estimation/2(EOLFric)

== system ES105A_StHlthSigNormn/call_StHlthSigNormnInit1/CopyRight2 ==

== system ES105A_StHlthSigNormn/call_UpdRawSig/CopyRight2 ==

== system ES105A_StHlthSigNormn/StHlthSigNormn/StHlthSigNormnInit1/CopyRight2 ==

== system ES105A_StHlthSigNormn/StHlthSigNormn/StHlthSigNormnInit1/GetFricLrngData ==
  note: Get NVM Data
  CopyRight2 : Subsystem  Description=|  mask(Copyright Information){none=on}
      | Copyright info block.                                               
      |                                                                     
      | Place copyright information at the top of every subsystem in design.
      mask prompts: none "No parameters"
      mask help: Place copyright information at the top of every subsystem in design.
      mask Display:
      | NxtrConf = 'Nexteer Confidential';
      | 
      | sys = bdroot; %handle for the current model ("system")
      | first = get_param(sys,'Created');
      | first = first(end-3:end);  %year is last four digits
      | 
      | last = get_param(sys,'LastModifiedDate');
      | if isempty(last)
      |     last = datestr(now,'yyyy');
      | else
      |     last = last(end-3:end);
      | end
      | 
      | if strcmp(first,last)
      |     fprintf('%s -- Copyright %s Nexteer',NxtrConf,first)
      | else
      |     fprintf('%s -- %s%s- %s Nexteer',NxtrConf,char(169),first,last)
      | end
  Ground : Ground
  EolFric : Outport
  wires:
  Ground/1 -> EolFric/1
